simulink model "CALCULATOR"  (R2019a)
settings: Solver=FixedStepAuto  StartTime=0.0  StopTime=10.0  FixedStep=0.2  RelTol=1e-3
settings Model: Creator=Admin  LastModifiedBy=Admin

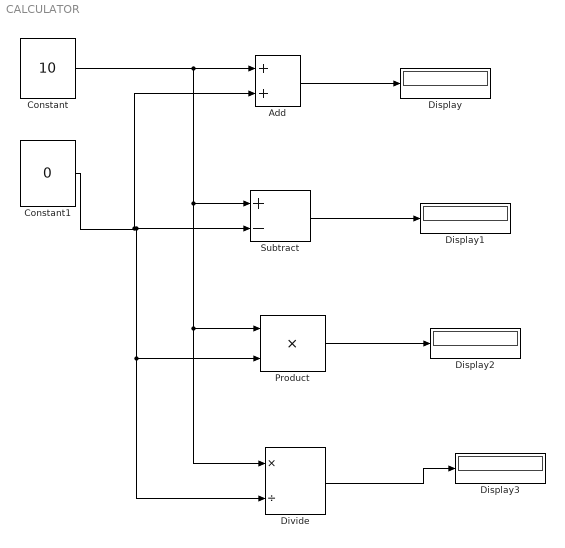
== system CALCULATOR ==
  Add : Sum
  Constant : Constant  Value=10
  Constant1 : Constant  Value=0
  Display{,1..3} (4 alike) : Display
  Divide : Product  Inputs=*/
  Product : Product
  Subtract : Sum  Inputs=+-
  wires:
  Divide/1 -> Display3/1
  Product/1 -> Display2/1
  Subtract/1 -> Display1/1
  Add/1 -> Display/1
  Constant/1 -> Add/1, Subtract/1, Product/1, Divide/1
  Constant1/1 -> Divide/2, Product/2, Subtract/2, Add/2
